simulink model "43_BusNetworkElectricityTransmissionModel"  (R2023b)
settings: Solver=VariableStepAuto  StartTime=0.0  StopTime=0.8  RelTol=1e-3
model workspace (MAT data in the model file):
  BESS_Fp_KDroop = 0.025
  BESS_KSI = 817
  BESS_PWM_fs = 560
  BESS_P_Ki = 0.5
  BESS_P_Kp = 0.0636
  BESS_Pnom = 3000000
  BESS_Q_Ki = 1
  BESS_Q_Kp = 0.0257
  BESS_Vd_Ki = 850
  BESS_Vd_Kp = 0.216
  BESS_Vnom = 1000
  BESS_Vq_KDroop = 0.025
  BESS_Vq_Ki = 850
  BESS_Vq_Kp = 0.216
  Compensation_Ki = 30
  Compensation_Kp = 3
  DC_Ki = 400
  DC_Kp = 8
  F = 0.01
  Flux_min = 0.5
  Grid_Freq_PWM = 2700
  Grid_Ireg_Ki = 5
  Grid_Ireg_Kp = 0.83
  Grid_Ireg_lim = 1.1
  Grid_Modindex_Upper = 1.1
  Grid_conv_Imax = 0.8
  H = 0.685
  Idref_max = 0.9
  Iqref_Tc = 0.3
  Ki_Var = 0.05
  Ki_Vreg = 20
  Ksh = 1.1
  L_pu = 0.3
  Llr = 0.16
  Lls = 0.18
  Lm = 2.9
  LowLoad_P = 130
  Nb_wt = 6
  P_mech = 1080000
  PeakShav_P = 200
  Pitch_Ki = 0
  Pitch_Kp = 150
  Pitch_Max = 27
  Pitch_Tc = 0.01
  Pitch_rate = 10
  Q_Filt = 50
  R_pu = 0.003
  Rotor_Freq_PWM = 1620
  Rotor_Ireg_Ki = 8
  Rotor_Ireg_Kp = 0.6
  Rotor_Ireg_lim = 0.1
  Rotor_Modindex_Upper = 2
  Rr = 0.016
  Rs = 0.023
  SOCBESS : Simulink.Parameter (value not decoded)
  T_set = 0.0001
  Tp = 5e-05
  Ts = 5e-06
  Var_C_Filt = 720000
  Var_reg_max = 1.1
  Var_reg_min = 0.9
  WT_Coeff = [0.645 116 0.4 5 21 0.00912 0.08 0.035]
  WT_H = 4.32
  WT_IGBTRon = 5.931
  WT_Param = [91.204 10143]
  Wind_Freq_Filt = 10000
  Wind_Freq_nom = 60
  Wind_P_nom = 1200000
  Wind_Rotor_V_nom = 1950
  Wind_V_nom = 500
  Zeta_Filt = 0.707106781187
  init = [-0.2 0 0 0 0 0 0 0]
  p = 3
  torque0 = 0.83
  v_Ki = 0.1
  v_Kp = 3.6
  v_Max = 1.2
  v_Min = 0.7
  v_T = 5
  vreg_max = 1
  wind_VDC_nom = 1150
  wt0 = 1.2
undefined symbols (not defined in the file): D1, D11, Delta, DiscIntNeverNeededParam, Iabc, Ion, Lithium, P, Q, Vabc
libraries: powerlib_extras x156, spsSeriesRLCBranchLib x66, spsLoadFlowBusLib x43, spsThreePhaseSeriesRLCLoadLib x33, spsThreePhaseTransformerTwoWindingsLib x32, spsThreePhaseVIMeasurementLib x30, simulink_extras x30, spsDistributedParametersLineLib x22, spsGenericPowerSystemStabilizerLib x20, spsSynchronousMachinepuStandardLib x10, spsExcitationSystemLib x10, spsHydraulicTurbineandGovernorLib x10
(part 3 of 19)

== system 43_BusNetworkElectricityTransmissionModel/North Network ==
  1320 MVar : spsThreePhaseSeriesRLCLoadLib/Three-Phase Series RLC Load  LConnTagsString=A|B|C  Configuration=Y (grounded)  NominalVoltage=650e3  Vabc=[1e3 1e3 1e3]  Vabcp=[1e3 1e3 1e3]  NominalFrequency=60  UnbalancedPower=off  ActivePower=4400e3  InductivePower=1320e6  CapacitivePower=0  Pabc=[10e3 9e3 11e3]  QLabc=[100 90 110]  QCabc=[100 90 110]  Pabcp=[10e3 9e3 11e3]  QLabcp=[100 90 110]  QCabcp=[100 90 110]  Measurements=None  LoadType=constant Z
  135 MW : spsThreePhaseSeriesRLCLoadLib/Three-Phase Series RLC Load  LConnTagsString=A|B|C  Configuration=Y (grounded)  NominalVoltage=17e3  Vabc=[1e3 1e3 1e3]  Vabcp=[1e3 1e3 1e3]  NominalFrequency=60  UnbalancedPower=off  ActivePower=135e6  InductivePower=0  CapacitivePower=0  Pabc=[10e3 9e3 11e3]  QLabc=[100 90 110]  QCabc=[100 90 110]  Pabcp=[10e3 9e3 11e3]  QLabcp=[100 90 110]  QCabcp=[100 90 110]  Measurements=None  LoadType=constant Z
  155 MW : spsThreePhaseSeriesRLCLoadLib/Three-Phase Series RLC Load  LConnTagsString=A|B|C  Configuration=Y (grounded)  NominalVoltage=17e3  Vabc=[1e3 1e3 1e3]  Vabcp=[1e3 1e3 1e3]  NominalFrequency=60  UnbalancedPower=off  ActivePower=155e6  InductivePower=0  CapacitivePower=0  Pabc=[10e3 9e3 11e3]  QLabc=[100 90 110]  QCabc=[100 90 110]  Pabcp=[10e3 9e3 11e3]  QLabcp=[100 90 110]  QCabcp=[100 90 110]  Measurements=None  LoadType=constant Z
  1980 MVar : spsThreePhaseSeriesRLCLoadLib/Three-Phase Series RLC Load  LConnTagsString=A|B|C  Configuration=Y (grounded)  NominalVoltage=650e3  Vabc=[1e3 1e3 1e3]  Vabcp=[1e3 1e3 1e3]  NominalFrequency=60  UnbalancedPower=off  ActivePower=6600e3  InductivePower=1980e6  CapacitivePower=0  Pabc=[10e3 9e3 11e3]  QLabc=[100 90 110]  QCabc=[100 90 110]  Pabcp=[10e3 9e3 11e3]  QLabcp=[100 90 110]  QCabcp=[100 90 110]  Measurements=None  LoadType=constant Z
  205 MW : spsThreePhaseSeriesRLCLoadLib/Three-Phase Series RLC Load  LConnTagsString=A|B|C  Configuration=Y (grounded)  NominalVoltage=17e3  Vabc=[1e3 1e3 1e3]  Vabcp=[1e3 1e3 1e3]  NominalFrequency=60  UnbalancedPower=off  ActivePower=205e6  InductivePower=0  CapacitivePower=0  Pabc=[10e3 9e3 11e3]  QLabc=[100 90 110]  QCabc=[100 90 110]  Pabcp=[10e3 9e3 11e3]  QLabcp=[100 90 110]  QCabcp=[100 90 110]  Measurements=None  LoadType=constant Z
  "2700 MVA 17KV :650KV Transformer " : spsThreePhaseTransformerTwoWindingsLib/Three-Phase Transformer (Two Windings)  Winding1Connection=Yg  Winding2Connection=Delta (D1)  CoreType=Three single-phase transformers  SetSaturation=off  Hysteresis=off  DataFile='hysteresis'  SetInitialFlux=off  Measurements=None  UNITS=pu  NominalPower=[ 2700e6 , 60 ]  Winding1=[650e3 , 0.002 , 0.08 ]  Winding2=[17e3 , 0.002 , 0.08 ]  Rm=500  Lm=500  L0=0.5  Saturation=[ 0,0 ; 0.0024,1.2 ; 1.0,1.52 ]  InitialFluxes=[ 0.8 , -0.8 , 0.7 ]  BreakLoop=off  DiscreteSolver=Trapezoidal iterative  DataType=off  TransfoNumber=1
  "3100 MVA 17KV :650KV Transformer " : spsThreePhaseTransformerTwoWindingsLib/Three-Phase Transformer (Two Windings)  Winding1Connection=Yg  Winding2Connection=Delta (D1)  CoreType=Three single-phase transformers  SetSaturation=off  Hysteresis=off  DataFile='hysteresis'  SetInitialFlux=off  Measurements=None  UNITS=pu  NominalPower=[ 3100e6 , 60 ]  Winding1=[ 650e3 , 0.002 , 0.08 ]  Winding2=[ 17e3 , 0.002 , 0.08 ]  Rm=500  Lm=500  L0=0.5  Saturation=[ 0,0 ; 0.0024,1.2 ; 1.0,1.52 ]  InitialFluxes=[ 0.8 , -0.8 , 0.7 ]  BreakLoop=off  DiscreteSolver=Trapezoidal iterative  DataType=off  TransfoNumber=1
  "4100 MVA 17KV :650KV Transformer " : spsThreePhaseTransformerTwoWindingsLib/Three-Phase Transformer (Two Windings)  Winding1Connection=Yg  Winding2Connection=Delta (D1)  CoreType=Three single-phase transformers  SetSaturation=off  Hysteresis=off  DataFile='hysteresis'  SetInitialFlux=off  Measurements=None  UNITS=pu  NominalPower=[ 4100e6 , 60 ]  Winding1=[ 650e3 , 0.002 , 0.08 ]  Winding2=[ 17e3 , 0.002 , 0.08 ]  Rm=500  Lm=500  L0=0.5  Saturation=[ 0,0 ; 0.0024,1.2 ; 1.0,1.52 ]  InitialFluxes=[ 0.8 , -0.8 , 0.7 ]  BreakLoop=off  DiscreteSolver=Trapezoidal iterative  DataType=off  TransfoNumber=1
  660 MVar : spsThreePhaseSeriesRLCLoadLib/Three-Phase Series RLC Load  LConnTagsString=A|B|C  Configuration=Y (grounded)  NominalVoltage=650e3  Vabc=[1e3 1e3 1e3]  Vabcp=[1e3 1e3 1e3]  NominalFrequency=60  UnbalancedPower=off  ActivePower=2200e3  InductivePower=660e6  CapacitivePower=0  Pabc=[10e3 9e3 11e3]  QLabc=[100 90 110]  QCabc=[100 90 110]  Pabcp=[10e3 9e3 11e3]  QLabcp=[100 90 110]  QCabcp=[100 90 110]  Measurements=None  LoadType=constant Z
  990 Mvar : spsThreePhaseParallelRLCLoadLib/Three-Phase Parallel RLC Load  LConnTagsString=A|B|C  Configuration=Y (grounded)  NominalVoltage=650e3  Vabc=[1e3 1e3 1e3]  Vabcp=[1e3 1e3 1e3]  NominalFrequency=60  UnbalancedPower=off  ActivePower=3300e3  InductivePower=990e6  CapacitivePower=0  Pabc=[10e3 9e3 11e3]  QLabc=[100 90 110]  QCabc=[100 90 110]  Pabcp=[10e3 9e3 11e3]  QLabcp=[100 90 110]  QCabcp=[100 90 110]  Measurements=None  LoadType=constant Z
  ATL-CAD 447 km : spsDistributedParametersLineLib/Distributed Parameters Line  Phases=3  Length=447  Frequency=60  Resistance=[0.01273 0.3864]/6  Inductance="[0.9337e-3  4.1264e-3]/6"  Capacitance=[12.74e-9 7.751e-9]*6  x1=[-0.00258 -1.67008857282466e-09 -194881.82529365 -120209.574728766;-0.00252 -2.05415012980081e-09 -192113.110957955 -124586.590676799;-0.00246 -2.43716074561422e-09 -189246.108004852 -128899.865822947;-0.0024 -2.81892446495662e-09 -186282.283246028 -133147.193415944;-0.00234 -3.19924597045502e-09 -183223.153028994 -137326.400444512;-0.00228 -3.57793068259966e-09 -180070.282461296 -141435.348749113;-0.00222 -3.95478485929453e-09 -176825.284609774 -145471.936115869;-0.00216 -4.32961569497935e-09 -173489.819675291 -149434.097352096;-0.0021 -4.70223141927253e-09 -170065.594143338 -153319.805342892;-0.00204 -5.07244139508436e-09 -166554.359910971 -157127.072088251;-0.00198 -5.44005621615053e-09 -162957.913390503 -160853.949720156;-0.00192 -5.80488780393583e-09 -159278.094590428 -164498.531499144;-0.00186 -6.16674950385864e-09 -155516.78617404 -168058.952789834;-0.0018 -6.52545618078685e-09 -151675.912496225 -171533.392014904;-0.00174 -6.88082431375641e-09 -147757.438618928 -174920.071587046;-0.00168 -7.23267208986403e-09 -143763.369305791 -178217.258818414;-0.00162 -7.58081949728606e-09 -139695.747996475 -181423.266807093;-0.00156 -7.92508841737585e-09 -135556.655761204 -184536.455300158;-0.0015 -8.2653027157925e-09 -131348.210236046 -187555.231532849;-0.00144 -8.60128833261452e-09 -127072.564539495 -190478.051043466;-0.00138 -8.93287337139205e-09 -122731.906170895 -193303.41846354;-0.00132 -9.25988818709224e-09 -118328.455891273 -196029.88828289;-0.00126 -9.58216547289286e-09 -113864.466587159 -198656.06558918;-0.0012 -9.89954034577949e-09 -109342.222117965 -201180.606781572;-0.00114 -1.02118504309027e-08 -104764.036147524 -203602.220258145;-0.00108 -1.05189359446522e-08 -100132.250960373 -205919.667076697;-0.00102 -1.08206397764049e-08 -95449.2362633992 -208131.761588614;-0.00096 -1.11168075689055e-08 -90717.387973454 -210237.37204547;-0.0009 -1.14072877972388e-08 -85939.126991557 -212235.421178048;-0.00084 -1.16919318463526e-08 -81116.8979643186 -214124.886747491;-0.00078 -1.19705940870918e-08 -76253.1680332137 -215904.802068301;-0.00072 -1.22431319507049e-08 -71350.4255723465 -217574.256502911;-0.00066 -1.25094060017849e-08 -66411.1789153522 -219132.395927584;-0.0006 -1.27692800096072e-08 -61437.9550720873 -220578.423169399;-0.00054 -1.30226210178274e-08 -56433.2984357647 -221911.598414101;-0.00048 -1.32692994125045e-08 -51399.7694811948 -223131.239584599;-0.00042 -1.35091889884137e-08 -46339.9434547999 -224236.722689934;-0.00036 -1.37421670136153e-08 -41256.4090570697 -225227.482144522;-0.0003 -1.39681142922467e-08 -36151.7671181352 -226103.01105752;-0.00024 -1.41869152255051e-08 -31028.6292671352 -226862.861492158;-0.00018 -1.43984578707901e-08 -25889.616596059 -227506.644694913;-0.00012 -1.46026339989755e-08 -20737.3583187471 -228034.031294402;-6e-05 -1.47993391497814e-08 -15574.490425737 -228444.751469897]  x2=[-0.00258 5.15041171457139e-09 -301593.332748427 -116993.562625722;-0.00252 4.92493877262698e-09 -298870.048576722 -123784.957337496;-0.00246 4.69694614100409e-09 -295993.856965682 -130513.021377814;-0.0024 4.46655046494587e-09 -292966.22942808 -137174.312544791;-0.00234 4.23386961913743e-09 -289788.714954109 -143765.422798781;-0.00228 3.99902264739891e-09 -286462.939218889 -150282.980005987;-0.00222 3.76212970178055e-09 -282990.603750737 -156723.649663712;-0.00216 3.52331198109059e-09 -279373.485060641 -163084.136606349;-0.0021 3.28269166888779e-09 -275613.43373336 -169361.186691249;-0.00204 3.04039187097001e-09 -271712.37348063 -175551.588463604;-0.00198 2.79653655239106e-09 -267672.30015696 -181652.17479948;-0.00192 2.55125047403786e-09 -263495.280738514 -187659.824526183;-0.00186 2.30465912880045e-09 -259183.45226561 -193571.464019103;-0.0018 2.05688867736754e-09 -254739.020749366 -199384.068774241;-0.00174 1.80806588368036e-09 -250164.260043072 -205094.664955601;-0.00168 1.55831805007787e-09 -245461.510678835 -210700.330916655;-0.00162 1.30777295216655e-09 -240633.178670128 -216198.198695118;-0.00156 1.05655877344804e-09 -235681.734280824 -221585.455480246;-0.0015 8.04804039738072e-10 -230609.710761363 -226859.345051921;-0.00144 5.52637553410304e-10 -225419.7030527 -232017.169190789;-0.00138 3.00188327498644e-10 -220114.366458677 -237056.289058714;-0.00132 4.75855196917949e-11 -214696.415287529 -241974.126548861;-0.00126 -2.05041633746211e-10 -209168.621463186 -246768.165604697;-0.0012 -4.57563884095657e-10 -203533.81310711 -251435.953507259;-0.00114 -7.0985203630719e-10 -197794.873091376 -255975.102130004;-0.00108 -9.61777015100393e-10 -191954.73756374 -260383.289160623;-0.00102 -1.21320993100107e-09 -186016.394445451 -264658.259289177;-0.00096 -1.46402214628351e-09 -179982.881902575 -268797.825361957;-0.0009 -1.71408534078389e-09 -173857.286791617 -272799.869500469;-0.00084 -1.96327157755127e-09 -167642.743080223 -276662.344184983;-0.00078 -2.21145336830249e-09 -161342.430243787 -280383.273302079;-0.00072 -2.45850373864752e-09 -154959.571638773 -283960.753155667;-0.00066 -2.70429629305194e-09 -148497.432853586 -287392.953440949;-0.0006 -2.94870527950318e-09 -141959.320037833 -290678.118180839;-0.00054 -3.19160565384762e-09 -135348.578210842 -293814.566624354;-0.00048 -3.43287314376546e-09 -128668.589550285 -296800.694106514;-0.00042 -3.67238431235074e-09 -121922.771661791 -299634.972869324;-0.00036 -3.91001662126397e-09 -115114.575830441 -302315.952843396;-0.0003 -4.14564849342495e-09 -108247.485255024 -304842.262389837;-0.00024 -4.37915937521393e-09 -101325.013265967 -307212.609002002;-0.00018 -4.61042979814898e-09 -94350.7015278514 -309425.779966765;-0.00012 -4.83934144000835e-09 -87328.118227434 -311480.642984966;-6e-05 -5.06577718536627e-09 -80260.8562480934 -313376.146750715]  x3=[-0.00258 5.51282931221187e-12 -5052.77243318941 2918.73418538423;-0.00252 4.31538249983226e-12 -5117.49377650402 2803.70636456851;-0.00246 3.11572785802664e-12 -5179.59691544217 2687.24411577014;-0.0024 1.91447915227681e-12 -5239.05007689043 2569.40702322757;-0.00234 7.12250963617166e-13 -5295.82284351283 2450.25537457474;-0.00228 -4.90341625796339e-13 -5349.88616931294 2329.85012999677;-0.00222 -1.69268334737362e-12 -5401.2123944943 2208.2528910416;-0.00216 -2.89415906087319e-12 -5449.77525961171 2085.52586910356;-0.0021 -4.09415406911931e-12 -5495.54991900603 1961.7318535948;-0.00204 -5.29205443249241e-12 -5538.5129535157 1836.9341798211;-0.00198 -6.48724728303191e-12 -5578.6423824584 1711.19669657837;-0.00192 -7.67912113799086e-12 -5615.91767487677 1584.58373348638;-0.00186 -8.86706621268178e-12 -5650.31976004245 1457.1600680766;-0.0018 -1.00504747324537e-11 -5681.83103721298 1328.99089265078;-0.00174 -1.12287412436412e-11 -5710.43538463672 1200.14178092734;-0.00168 -1.2401262923325e-11 -5736.11816780095 1070.67865449271;-0.00162 -1.35674398877484e-11 -5758.86624691927 940.66774907458;-0.00156 -1.47266754992277e-11 -5778.66798365404 810.175580654477;-0.0015 -1.58783766714039e-11 -5795.51324707088 679.268911436989;-0.00144 -1.70219541726763e-11 -5809.39341882173 548.014715692963;-0.00138 -1.81568229276645e-11 -5820.30139755427 416.480145494241;-0.00132 -1.92824023165433e-11 -5828.23160254502 284.732496357416;-0.00126 -2.03981164720992e-11 -5833.17997655457 152.839172814202;-0.0012 -2.15033945743541e-11 -5835.14398790334 20.8676539260338;-0.00114 -2.25976711426077e-11 -5834.12263176683 -111.114541239473;-0.00108 -2.36803863247478e-11 -5830.11643068972 -243.039888152521;-0.00102 -2.4750986183681e-11 -5823.12743431851 -374.840891367929;-0.00096 -2.58089229807369e-11 -5813.15921835287 -506.450119057049;-0.0009 -2.68536554559018e-11 -5800.2168827163 -637.800237507139;-0.00084 -2.7884649104737e-11 -5784.30704894683 -768.824045570526;-0.00078 -2.89013764518411e-11 -5765.43785680943 -899.454509045965;-0.00072 -2.99033173207164e-11 -5743.61896013143 -1029.62479497457;-0.00066 -3.08899590999007e-11 -5718.86152186356 -1159.26830583278;-0.0006 -3.18607970052286e-11 -5691.17820836869 -1288.31871360492;-0.00054 -3.28153343380888e-11 -5660.58318294154 -1416.70999371778;-0.00048 -3.3753082739544e-11 -5627.09209856244 -1544.37645882006;-0.00042 -3.46735624401844e-11 -5590.72208988901 -1671.25279238922;-0.00036 -3.55763025055866e-11 -5551.49176448973 -1797.27408214859;-0.0003 -3.64608410772525e-11 -5509.42119332396 -1922.37585327772;-0.00024 -3.73267256089044e-11 -5464.53190047329 -2046.4941013989;-0.00018 -3.81735130980161e-11 -5416.8468521294 -2169.56532532294;-0.00012 -3.90007703124615e-11 -5366.39044484413 -2291.52655953759;-6e-05 -3.98080740121637e-11 -5313.18849304779 -2412.31540642183]  x4=[-0.00258 1.21970167270157e-10 -7329.45055634832 -4834.93116395816;-0.00252 1.19241005783673e-10 -7218.22081108888 -4999.4692217727;-0.00246 1.1645083839531e-10 -7103.29809068509 -5161.44945875382;-0.0024 1.1360109260626e-10 -6984.74119172425 -5320.78900281922;-0.00234 1.10693226399125e-10 -6862.61077010654 -5477.40633291389;-0.00228 1.0772872749199e-10 -6736.96931001239 -5631.22132071782;-0.00222 1.04709112577271e-10 -6607.88109193435 -5782.15527164106;-0.00216 1.01635926545756e-10 -6475.41215979007 -5930.13096508538;-0.0021 9.85107416962035e-11 -6339.63028713298 -6075.07269395175;-0.00204 9.53351569309305e-11 -6200.6049424781 -6216.90630337345;-0.00198 9.21107969377804e-11 -6058.40725376064 -6355.55922865513;-0.00192 8.88393113589052e-11 -5913.10997194567 -6490.96053239819;-0.00186 8.5522373946777e-11 -5764.78743380733 -6623.04094079372;-0.0018 8.21616817078658e-11 -5613.51552389683 -6751.73287906421;-0.00174 7.87589540344196e-11 -5459.37163571847 -6876.9705060361;-0.00168 7.53159318247913e-11 -5302.43463213369 -6998.68974782529;-0.00162 7.18343765927629e-11 -5142.78480501338 -7116.82833061858;-0.00156 6.8316069566323e-11 -4980.50383415909 -7231.32581253405;-0.0015 6.47628107763572e-11 -4815.67474551411 -7342.1236145443;-0.00144 6.11764181357191e-11 -4648.38186868589 -7449.16505044649;-0.00138 5.75587265091524e-11 -4478.71079380142 -7552.39535586414;-0.00132 5.39115867745408e-11 -4306.74832771779 -7651.76171626551;-0.00126 5.02368648759636e-11 -4132.58244961014 -7747.21329398453;-0.0012 4.65364408690454e-11 -3956.30226595993 -7838.70125423031;-0.00114 4.2812207959084e-11 -3777.99796496638 -7926.17879007188;-0.00108 3.90660715324522e-11 -3597.76077040459 -8009.6011463855;-0.00102 3.52999481817663e-11 -3415.68289495368 -8088.92564275222;-0.00096 3.15157647253225e-11 -3231.85749301915 -8164.11169529394;-0.0009 2.7715457221301e-11 -3046.37861307333 -8235.12083743692;-0.00084 2.39009699772422e-11 -2859.34114953846 -8301.91673959193;-0.00078 2.00742545553039e-11 -2670.84079423694 -8364.46522774117;-0.00072 1.62372687738056e-11 -2480.97398743362 -8422.73430092236;-0.00066 1.23919757055724e-11 -2289.8378684952 -8476.69414760096;-0.0006 8.54034267359075e-12 -2097.53022619192 -8526.31716092235;-0.00054 4.68434024448995e-12 -1904.14944866701 -8571.57795283598;-0.00048 8.25941220363423e-13 -1709.79447309954 -8612.4533670844;-0.00042 -3.03288037055309e-12 -1514.56473508625 -8648.92249105037;-0.00036 -6.89015028383084e-12 -1318.56011776856 -8680.9666664562;-0.0003 -1.0743895068908e-11 -1121.88090073043 -8708.56949890966;-0.00024 -1.45921430787436e-11 -924.627708693503 -8731.71686629162;-0.00018 -1.84329254785483e-11 -726.901460035657 -8750.3969259812;-0.00012 -2.22642772530769e-11 -528.803315159263 -8764.6001209147;-6e-05 -2.60842382119663e-11 -330.434624735671 -8774.31918447516]  x5=0.00252797080447097  V1=[6.404e-19 2.341e-08 2.341e-08;377 377 377;-1.588 0.8733 -0.6975]  V2=[3.447e-16 8.016e-05 8.016e-05;377 377 377;2.581 0.8892 -0.6816]  I1=[4.995e-19 5.332e-07 5.332e-07;377 377 377;1.203 -0.6479 -2.219]  I2=[4.022e-19 5.225e-07 5.225e-07;377 377 377;-2.95 1.909 0.3385]  nHarmo=1  Measurements=None  Decoupling=off  VsMag0=0  VrMag0=0  VsAngle0=0  VrAngle0=0  IsMag0=0  IrMag0=0  IsAngle0=0  IrAngle0=0
      settings: LibrarySourceBlock=sps_lib/Power Grid Elements/Distributed Parameters Line
  BMW 1 : spsThreePhaseVIMeasurementLib/Three-Phase V-I Measurement  VoltageMeasurement=no  SetLabelV=off  LabelV=Vabc  Vpu=off  VpuLL=off  CurrentMeasurement=no  SetLabelI=off  LabelI=Iabc  Ipu=off  Pbase=100e6  Vbase=500e3  OutputType=Complex  PhasorSimulation=off  PSBequivalent=0
  BMW- FER 131 km : spsDistributedParametersLineLib/Distributed Parameters Line  Phases=3  Length=131  Frequency=60  Resistance=[0.01273 0.3864]/6  Inductance="[0.9337e-3  4.1264e-3]/6"  Capacitance=[12.74e-9 7.751e-9]*6  x1=[-0.00078 -1.19705940870918e-08 -76253.1680332137 -215904.802068301;-0.00072 -1.22431319507049e-08 -71350.4255723465 -217574.256502911;-0.00066 -1.25094060017849e-08 -66411.1789153522 -219132.395927584;-0.0006 -1.27692800096072e-08 -61437.9550720873 -220578.423169399;-0.00054 -1.30226210178274e-08 -56433.2984357647 -221911.598414101;-0.00048 -1.32692994125045e-08 -51399.7694811948 -223131.239584599;-0.00042 -1.35091889884137e-08 -46339.9434547999 -224236.722689934;-0.00036 -1.37421670136153e-08 -41256.4090570697 -225227.482144522;-0.0003 -1.39681142922467e-08 -36151.7671181352 -226103.01105752;-0.00024 -1.41869152255051e-08 -31028.6292671352 -226862.861492158;-0.00018 -1.43984578707901e-08 -25889.616596059 -227506.644694913;-0.00012 -1.46026339989755e-08 -20737.3583187471 -228034.031294402;-6e-05 -1.47993391497814e-08 -15574.490425737 -228444.751469897]  x2=[-0.00078 -1.84679215935695e-10 -40323.6266116141 -194988.996299748;-0.00072 2.82824148749058e-10 -35903.1411858874 -195851.159993976;-0.00066 7.50182815373322e-10 -31464.2870497162 -196613.122615838;-0.0006 1.21715767460746e-09 -27009.3352028971 -197274.494331177;-0.00054 1.68350981348478e-09 -22540.5648811132 -197834.936770003;-0.00048 2.14900063763383e-09 -18060.2623898343 -198294.163199608;-0.00042 2.6133919933477e-09 -13570.7199346015 -198651.938671265;-0.00036 3.07644628942785e-09 -9074.23444829206 -198908.080140432;-0.0003 3.53792661874013e-09 -4573.10641596632 -199062.456560401;-0.00024 3.9975968794209e-09 -69.6386978968809 -199114.988949342;-0.00018 4.45522189567106e-09 4433.86464861718 -199065.650430714;-0.00012 4.91056753807636e-09 8935.09954804861 -198914.466247016;-6e-05 5.36340084339233e-09 13431.7630854496 -198661.513746869]  x3=[-0.00078 -8.93963344042616e-10 801.480589851872 -9198.62669723828;-0.00072 -8.84038389071924e-10 1009.32547419504 -9178.14688538209;-0.00066 -8.73661143726232e-10 1216.65396897542 -9152.97136398669;-0.0006 -8.62836917196007e-10 1423.36000110408 -9123.11301331401;-0.00054 -8.51571247355552e-10 1629.33781595552 -9088.58710944798;-0.00048 -8.39869897929723e-10 1834.48203147361 -9049.41131647897;-0.00042 -8.27738855545101e-10 2038.68769208707 -9005.60567746655;-0.00036 -8.15184326667126e-10 2241.85032240664 -8957.19260418508;-0.0003 -8.02212734424755e-10 2443.86598067664 -8904.19686565742;-0.00024 -7.88830715324265e-10 2644.63131195347 -8846.64557548264;-0.00018 -7.75045115853899e-10 2844.04360098393 -8784.56817796424;-0.00012 -7.60862988981075e-10 3042.00082475626 -8717.99643304583;-6e-05 -7.46291590543957e-10 3238.40170469692 -8646.96440006223]  x4=[-0.00078 7.88145612187523e-10 -4148.32191911194 353.877291066962;-0.00072 7.79406939715943e-10 -4155.2640953326 259.961667664255;-0.00066 7.7026950825222e-10 -4160.08036166163 165.913043068831;-0.0006 7.60737992675131e-10 -4162.76825400819 71.7795342948529;-0.00054 7.50817269484168e-10 -4163.32639719688 -22.3906982152036;-0.00048 7.40512414304629e-10 -4161.75450567134 -116.549475230321;-0.00042 7.29828699290835e-10 -4158.05338364032 -210.648623380323;-0.00036 7.187715904288e-10 -4152.22492466623 -304.639999802266;-0.0003 7.0734674473973e-10 -4144.27211069639 -398.475516771209;-0.00024 6.95560007385786e-10 -4134.19901053738 -492.107166302792;-0.00018 6.83417408679592e-10 -4122.01077777336 -585.487044714998;-0.00012 6.70925160999016e-10 -4107.71364812942 -678.567377136572;-6e-05 6.58089655608801e-10 -4091.31493628129 -771.30054194952]  x5=0.000740859452764423  V1=[1.271e-18 2.341e-08 2.341e-08;377 377 377;2.226 1.284 -0.2866]  V2=[3.351e-20 3.07e-09 3.07e-09;377 377 377;-0.6702 -1.817 2.896]  I1=[5.66e-21 5.705e-10 5.705e-10;377 377 377;-2.518 2.745 1.174]  I2=[6.071e-21 5.74e-10 5.74e-10;377 377 377;0.8934 -0.2657 -1.836]  nHarmo=1  Measurements=None  Decoupling=off  VsMag0=0  VrMag0=0  VsAngle0=0  VrAngle0=0  IsMag0=0  IrMag0=0  IsAngle0=0  IrAngle0=0
      settings: LibrarySourceBlock=sps_lib/Power Grid Elements/Distributed Parameters Line
  BMW- ORE 215 km : spsDistributedParametersLineLib/Distributed Parameters Line  Phases=3  Length=215  Frequency=60  Resistance=[0.01273 0.3864]/6  Inductance="[0.9337e-3  4.1264e-3]/6"  Capacitance=[12.74e-9 7.751e-9]*6  x1=[-0.00126 -9.58216547289286e-09 -113864.466587159 -198656.06558918;-0.0012 -9.89954034577949e-09 -109342.222117965 -201180.606781572;-0.00114 -1.02118504309027e-08 -104764.036147524 -203602.220258145;-0.00108 -1.05189359446522e-08 -100132.250960373 -205919.667076697;-0.00102 -1.08206397764049e-08 -95449.2362633992 -208131.761588614;-0.00096 -1.11168075689055e-08 -90717.387973454 -210237.37204547;-0.0009 -1.14072877972388e-08 -85939.126991557 -212235.421178048;-0.00084 -1.16919318463526e-08 -81116.8979643186 -214124.886747491;-0.00078 -1.19705940870918e-08 -76253.1680332137 -215904.802068301;-0.00072 -1.22431319507049e-08 -71350.4255723465 -217574.256502911;-0.00066 -1.25094060017849e-08 -66411.1789153522 -219132.395927584;-0.0006 -1.27692800096072e-08 -61437.9550720873 -220578.423169399;-0.00054 -1.30226210178274e-08 -56433.2984357647 -221911.598414101;-0.00048 -1.32692994125045e-08 -51399.7694811948 -223131.239584599;-0.00042 -1.35091889884137e-08 -46339.9434547999 -224236.722689934;-0.00036 -1.37421670136153e-08 -41256.4090570697 -225227.482144522;-0.0003 -1.39681142922467e-08 -36151.7671181352 -226103.01105752;-0.00024 -1.41869152255051e-08 -31028.6292671352 -226862.861492158;-0.00018 -1.43984578707901e-08 -25889.616596059 -227506.644694913;-0.00012 -1.46026339989755e-08 -20737.3583187471 -228034.031294402;-6e-05 -1.47993391497814e-08 -15574.490425737 -228444.751469897]  x2=[-0.00126 6.50309734918414e-09 -202799.306931214 -207001.083285656;-0.0012 5.98047046812839e-09 -198065.563080492 -211534.981265528;-0.00114 5.45478386787474e-09 -193230.485227868 -215960.654040268;-0.00108 4.92630649940148e-09 -188296.547088512 -220275.837353906;-0.00102 4.39530874149545e-09 -183266.272956345 -224478.323478925;-0.00096 3.8620622624213e-09 -178142.236412563 -228565.962345769;-0.0009 3.32683988093099e-09 -172927.059008942 -232536.662642864;-0.00084 2.78991542668466e-09 -167623.408926607 -236388.392886568;-0.00078 2.25156360015433e-09 -162233.999610941 -240119.182460515;-0.00072 1.71205983208205e-09 -156761.588383335 -243727.122623823;-0.00066 1.17168014256445e-09 -151208.97503049 -247210.367487638;-0.0006 6.30700999835754e-10 -145579.000371999 -250567.134959523;-0.00054 8.93991788215252e-11 -139874.544806927 -253795.707655215;-0.00048 -4.51948380464494e-10 -134098.526840148 -256894.433777264;-0.00042 -9.93064714608022e-10 -128253.901589181 -259861.72796013;-0.00036 -1.53367297849383e-09 -122343.659272302 -262696.072081279;-0.0003 -2.07349658694482e-09 -116370.823678688 -265396.016037886;-0.00024 -2.61225935622812e-09 -110338.450621394 -267960.178488734;-0.00018 -3.14968564535578e-09 -104249.626373943 -270387.247560931;-0.00012 -3.68550049710776e-09 -98107.4660913263 -272675.981521095;-6e-05 -4.21942977870521e-09 -91915.1122162403 -274825.20941064]  x3=[-0.00126 1.65771973171058e-10 -4039.34540789377 3058.66441287293;-0.0012 1.6818222170819e-10 -4107.490998384 2966.52179794441;-0.00114 1.70506425113046e-10 -4173.53512058175 2872.86145564905;-0.00108 1.72743394280217e-10 -4237.44398509375 2777.7313043486;-0.00102 1.74891984734944e-10 -4299.18489496401 2681.18001438628;-0.00096 1.76951097218648e-10 -4358.72626240221 2583.25698318608;-0.0009 1.78919678251335e-10 -4416.03762494456 2484.01230998018;-0.00084 1.80796720670572e-10 -4471.08966103899 2383.49677017723;-0.00078 1.82581264146776e-10 -4523.8542050466 2281.7617893847;-0.00072 1.84272395674528e-10 -4574.3042616517 2178.85941709861;-0.00066 1.8586925003969e-10 -4622.41401967311 2074.84230007404;-0.0006 1.87371010262064e-10 -4668.15886526966 1969.76365539007;-0.00054 1.88776908013369e-10 -4711.51539453308 1863.67724322296;-0.00048 1.90086224010338e-10 -4752.46142546187 1756.63733934142;-0.00042 1.91298288382714e-10 -4790.97600931 1648.69870733815;-0.00036 1.92412481015967e-10 -4827.0394413047 1539.91657061175;-0.0003 1.93428231868559e-10 -4860.6332707278 1430.34658411344;-0.00024 1.94345021263584e-10 -4891.74031035543 1320.04480587294;-0.00018 1.95162380154648e-10 -4920.3446452513 1209.06766831812;-0.00012 1.95879890365838e-10 -4946.43164090915 1097.47194940319;-6e-05 1.96497184805673e-10 -4969.98795073996 985.31474356]  x4=[-0.00126 -1.20908843861436e-10 -4184.12959328111 -10998.5446924139;-0.0012 -1.29836564733162e-10 -3934.2992777039 -11090.3669013412;-0.00114 -1.38697858819266e-10 -3682.45610191872 -11176.5150736354;-0.00108 -1.47488192517956e-10 -3428.72891354783 -11256.9451342996;-0.00102 -1.56203068532086e-10 -3173.24752410915 -11331.6159338286;-0.00096 -1.64838028170054e-10 -2916.14264260226 -11400.4892692618;-0.0009 -1.73388653626954e-10 -2657.54580863529 -11463.529903728;-0.00084 -1.81850570244804e-10 -2397.58932512683 -11520.7055844737;-0.00078 -1.90219448750705e-10 -2136.40619061727 -11571.9870593643;-0.00072 -1.98491007471773e-10 -1874.13003122435 -11617.3480918495;-0.00066 -2.06661014525727e-10 -1610.89503227751 -11656.7654743871;-0.0006 -2.14725289985993e-10 -1346.83586966624 -11690.2190403157;-0.00054 -2.22679708020235e-10 -1082.08764093738 -11717.6916741728;-0.00048 -2.30520199001206e-10 -816.785796176738 -11739.1693204514;-0.00042 -2.38242751588845e-10 -551.066068710306 -11754.6409907908;-0.00036 -2.4584341478255e-10 -285.064405660592 -11764.0987695985;-0.0003 -2.53318299942589e-10 -18.9168983935577 -11767.5378181001;-0.00024 -2.60663582779593e-10 247.240287108239 -11764.9563768148;-0.00018 -2.67875505311138e-10 513.270979910676 -11756.3557664558;-0.00012 -2.74950377784396e-10 779.039073795634 -11741.7403872542;-6e-05 -2.8188458056388e-10 1044.40859689545 -11721.117716708]  x5=0.00121591436904085  V1=[1.271e-18 2.341e-08 2.341e-08;377 377 377;2.047 1.175 -0.3959]  V2=[2.813e-15 0.004697 0.004697;377 377 377;-0.9882 1.143 -0.4279]  I1=[7.991e-18 6.252e-05 6.252e-05;377 377 377;-2.327 -0.3924 -1.963]  I2=[7.132e-18 6.19e-05 6.19e-05;377 377 377;0.3426 2.469 0.8982]  nHarmo=1  Measurements=None  Decoupling=off  VsMag0=0  VrMag0=0  VsAngle0=0  VrAngle0=0  IsMag0=0  IrMag0=0  IsAngle0=0  IrAngle0=0
      settings: LibrarySourceBlock=sps_lib/Power Grid Elements/Distributed Parameters Line
  CAD 3 : spsThreePhaseVIMeasurementLib/Three-Phase V-I Measurement  VoltageMeasurement=no  SetLabelV=off  LabelV=Vabc  Vpu=off  VpuLL=off  CurrentMeasurement=no  SetLabelI=off  LabelI=Iabc  Ipu=off  Pbase=100e6  Vbase=500e3  OutputType=Complex  PhasorSimulation=off  PSBequivalent=0
  Cs BMW- MPP8 : Subsystem
  Cs BMWN : Subsystem
  Cs FER : Subsystem
  Cs LTNN : Subsystem
  Cs ORED : Subsystem
  FER-LTN 78 km : spsDistributedParametersLineLib/Distributed Parameters Line  Phases=3  Length=78  Frequency=60  Resistance=[0.01273 0.3864]/6  Inductance="[0.9337e-3  4.1264e-3]/6"  Capacitance=[12.74e-9 7.751e-9]*6  x1=[-0.00048 -1.16937399343794e-09 0 0;-0.00042 -7.96828963434923e-10 0 0;-0.00036 -4.23876261010511e-10 0 0;-0.0003 -5.07066956586323e-11 -25934.923705434 -220693.628977832;-0.00024 3.22488812175697e-10 -20936.7468426592 -221223.782464588;-0.00018 6.95519328774809e-10 -15927.8583533331 -221640.753776489;-0.00012 1.0681940048336e-09 -10910.8208773604 -221944.329583308;-6e-05 1.44032217310156e-09 -5888.20122381812 -222134.354570052]  x2=[-0.00048 7.78041349050393e-09 0 0;-0.00042 8.5731532508491e-09 0 0;-0.00036 9.36150682757748e-09 0 0;-0.0003 1.01450708844321e-08 -7150.14822079248 -204050.585017666;-0.00024 1.09234445355629e-08 -2533.20208774904 -204160.128306381;-0.00018 1.16962295506273e-08 2085.04007829069 -204165.219501008;-0.00012 1.24630305585321e-08 6702.21549929925 -204065.855996799;-6e-05 1.32234552497128e-08 11315.9619430157 -203862.088629959]  x3=[-0.00048 -7.75649349725857e-10 0 0;-0.00042 -7.58329745316695e-10 0 0;-0.00036 -7.40622165397507e-10 0 0;-0.0003 -7.22535669493377e-10 2958.82173994833 -8816.93119537568;-0.00024 -7.0407951098981e-10 3157.48156193806 -8747.75517282301;-0.00018 -6.85263132398528e-10 3354.52595801715 -8674.10363708399;-0.00012 -6.66096160526503e-10 3549.8541166316 -8596.01426964524;-6e-05 -6.46588401550711e-10 3743.36610428622 -8513.52702247006]  x4=[-0.00048 8.01840901977148e-10 0 0;-0.00042 7.94117538895057e-10 0 0;-0.00036 7.85987890606462e-10 0 0;-0.0003 7.77456116389647e-10 -4166.96813804089 -533.728222533507;-0.00024 7.68526581257949e-10 -4153.83015319847 -627.838614952894;-0.00018 7.59203853726542e-10 -4138.56699209571 -721.627793535747;-0.00012 7.49492703475093e-10 -4121.18646364787 -815.047774005279;-6e-05 7.39398098907514e-10 -4101.69746005446 -908.050760973279]  x5=0.000441122422256679  V1=[6.391e-24 5.815e-13 5.815e-13;377 377 377;2.579 1.39 -0.1804]  V2=[2.845e-25 1.398e-13 1.398e-13;377 377 377;-0.3188 -1.706 3.006]  I1=[5.031e-26 2.613e-14 2.613e-14;377 377 377;-2.041 2.924 1.353]  I2=[5.244e-26 2.622e-14 2.622e-14;377 377 377;1.254 -0.1553 -1.726]  nHarmo=1  Measurements=None  Decoupling=off  VsMag0=0  VrMag0=0  VsAngle0=0  VrAngle0=0  IsMag0=0  IrMag0=0  IsAngle0=0  IrAngle0=0
      settings: LibrarySourceBlock=sps_lib/Power Grid Elements/Distributed Parameters Line
  LTN 3 : spsThreePhaseVIMeasurementLib/Three-Phase V-I Measurement  VoltageMeasurement=no  SetLabelV=off  LabelV=Vabc  Vpu=off  VpuLL=off  CurrentMeasurement=no  SetLabelI=off  LabelI=Iabc  Ipu=off  Pbase=100e6  Vbase=500e3  OutputType=Complex  PhasorSimulation=off  PSBequivalent=0
  Load Flow Bus : spsLoadFlowBusLib/Load Flow Bus  LConnTagsString=a  Phases=single  Connectors=on one side  ID=BUS_13  Vbase=17e3  Vref=1  Vangle=0  VLF=1  VLFb=1  VLFc=1  angleLF=0  angleLFb=0  angleLFc=0
  Load Flow Bus1 : spsLoadFlowBusLib/Load Flow Bus  LConnTagsString=a  Phases=single  Connectors=on one side  ID=BUS_14  Vbase=650e3  Vref=1  Vangle=0  VLF=1  VLFb=1  VLFc=1  angleLF=0  angleLFb=0  angleLFc=0
  Load Flow Bus2 : spsLoadFlowBusLib/Load Flow Bus  LConnTagsString=a  Phases=single  Connectors=on one side  ID=BUS_15  Vbase=17e3  Vref=1  Vangle=0  VLF=1  VLFb=1  VLFc=1  angleLF=0  angleLFb=0  angleLFc=0
  Load Flow Bus3 : spsLoadFlowBusLib/Load Flow Bus  LConnTagsString=a  Phases=single  Connectors=on one side  ID=BUS_16  Vbase=650e3  Vref=1  Vangle=0  VLF=1  VLFb=1  VLFc=1  angleLF=0  angleLFb=0  angleLFc=0
  Load Flow Bus4 : spsLoadFlowBusLib/Load Flow Bus  LConnTagsString=a  Phases=single  Connectors=on one side  ID=BUS_17  Vbase=17e3  Vref=1  Vangle=0  VLF=1  VLFb=1  VLFc=1  angleLF=0  angleLFb=0  angleLFc=0
  Load Flow Bus6 : spsLoadFlowBusLib/Load Flow Bus  LConnTagsString=a  Phases=single  Connectors=on one side  ID=BUS_18  Vbase=650e3  Vref=1  Vangle=0  VLF=1  VLFb=1  VLFc=1  angleLF=0  angleLFb=0  angleLFc=0
  Load Flow Bus7 : spsLoadFlowBusLib/Load Flow Bus  LConnTagsString=a  Phases=single  Connectors=on one side  ID=BUS_19  Vbase=650e3  Vref=1  Vangle=0  VLF=1  VLFb=1  VLFc=1  angleLF=0  angleLFb=0  angleLFc=0
  Load Flow Bus8 : spsLoadFlowBusLib/Load Flow Bus  LConnTagsString=a  Phases=single  Connectors=on one side  ID=BUS_20  Vbase=650e3  Vref=1  Vangle=0  VLF=1  VLFb=1  VLFc=1  angleLF=0  angleLFb=0  angleLFc=0
  MPP7 2700 MVA 17KV : spsSynchronousMachinepuStandardLib/Synchronous Machine pu Standard  PresetModel=No  MechanicalLoad=Mechanical power Pm  ShowDetailedParameters=on  RotorType=Salient-pole  Units=per unit standard parameters  MeasurementBus=off  NominalParameters=[2700e6 17000 60]  Reactances1=[ 1.81, 0.3, 0.23, 1.76, 0.65, 0.25, 0.15 ]  Reactances2=[ 1.305, 0.296, 0.252, 0.474, 0.243, 0.18 ]  dAxisTimeConstants=Short-circuit  qAxisTimeConstants=Open-circuit  TimeConstants1="[ 4.4849  0.0681  0.1  ]"  TimeConstants2=[ 8.0, 0.03, 1.0, 0.07 ]  TimeConstants3="[  4.49  0.0681  0.0513  ]"  TimeConstants4=[ 8.0, 0.03, 0.3371, 0.0295 ]  TimeConstants5=[ 1.01, 0.053, 0.1 ]  TimeConstants6=[ 1.3201, 0.023, 1.0, 0.07 ]  TimeConstants7=[0.012 0.003 0.003]  TimeConstants8=[ 1.3201, 0.0231, 0.3371, 0.0295 ]  StatorResistance=2.8544e-3  Mechanical=[3.5 0 32]  PolePairs=20  InitialConditions=[0 -81.9543 0.907703 0.907703 0.907703 -8.76021 -128.76 111.24 1.25655]  SetSaturation=off  Saturation=[0.6404,0.7127,0.8441,0.9214,0.9956,1.082,1.19,1.316,1.457;0.7,0.7698,0.8872,0.9466,0.9969,1.046,1.1,1.151,1.201]  LoadFlowParameters=[1,0,0,0,0]  TsPowergui=0  TsBlock=-1  IterativeModel=Trapezoidal non iterative  IterativeDiscreteModel=Trapezoidal non iterative  BusType=PV  Pref=2200e6  Qref=0  Qmin=-inf  Qmax=inf  PLF=0  QLF=0
  MPP7-BMW 330 km : spsDistributedParametersLineLib/Distributed Parameters Line  Phases=3  Length=330  Frequency=60  Resistance=[0.01273 0.3864]/6  Inductance="[0.9337e-3  4.1264e-3]/6"  Capacitance=[12.74e-9 7.751e-9]*6  x1=[-0.00192 1.38989509065807e-07 0 0;-0.00186 1.40148907189762e-07 0 0;-0.0018 1.41236602543144e-07 0 0;-0.00174 1.42252038640913e-07 0 0;-0.00168 1.43194695967198e-07 0 0;-0.00162 1.44064092241093e-07 0 0;-0.00156 1.44859782663398e-07 0 0;-0.0015 1.45581360144192e-07 0 0;-0.00144 1.46228455511102e-07 0 0;-0.00138 1.46800737698181e-07 0 0;-0.00132 1.47297913915288e-07 0 0;-0.00126 1.47719729797884e-07 0 0;-0.0012 1.48065969537168e-07 0 0;-0.00114 1.48336455990492e-07 -132077.727810692 -207582.11422983;-0.00108 1.48531050771989e-07 -127348.938431694 -210516.312840008;-0.00102 1.48649654323373e-07 -122554.994982656 -213342.807414642;-0.00096 1.48692205964875e-07 -117698.350133629 -216060.151866882;-0.0009 1.4865868392629e-07 -112781.488633858 -218666.955953093;-0.00084 1.48549105358111e-07 -107806.92604054 -221161.885984138;-0.00078 1.48363526322759e-07 -102777.207431817 -223543.665507712;-0.00072 1.48102041765898e-07 -97694.906104667 -225811.0759614;-0.00066 1.47764785467858e-07 -92562.6222583596 -227962.957296118;-0.0006 1.47351929975193e-07 -87382.9816641442 -229998.208569611;-0.00054 1.46863686512403e-07 -82158.6343218576 -231915.788509722;-0.00048 1.46300304873863e-07 -76892.2531041349 -233714.716047121;-0.00042 1.45662073296032e-07 -71586.5323889187 -235394.070817238;-0.00036 1.44949318309977e-07 -66244.1866809652 -236952.993631143;-0.0003 1.44162404574319e-07 -60867.949223054 -238390.686915118;-0.00024 1.43301734688665e-07 -55460.5705976098 -239706.415118714;-0.00018 1.42367748987633e-07 -50024.8173194544 -240899.50509107;-0.00012 1.41360925315566e-07 -44563.470420406 -241969.346425311;-6e-05 1.40281778782058e-07 -39079.3240264523 -242915.391770841]  x2=[-0.00192 9.24024719193905e-08 0 0;-0.00186 9.23789280720258e-08 0 0;-0.0018 9.23081214580931e-08 0 0;-0.00174 9.21900883035645e-08 0 0;-0.00168 9.20248889963828e-08 0 0;-0.00162 9.18126080555661e-08 0 0;-0.00156 9.15533540879663e-08 0 0;-0.0015 9.12472597327035e-08 0 0;-0.00144 9.0894481593306e-08 0 0;-0.00138 9.04952001575885e-08 0 0;-0.00132 9.00496197053113e-08 0 0;-0.00126 8.95579682036672e-08 0 0;-0.0012 8.90204971906491e-08 0 0;-0.00114 8.84374816463587e-08 -71122.359287635 -183857.838140937;-0.00108 8.78092198523211e-08 -66945.7512982624 -185419.440441792;-0.00102 8.71360332388793e-08 -62734.8926255105 -186886.17873076;-0.00096 8.64182662207438e-08 -58491.9376224838 -188257.30259743;-0.0009 8.56562860207837e-08 -54219.0570633627 -189532.110549496;-0.00084 8.48504824821492e-08 -49918.437032795 -190709.950371654;-0.00078 8.40012678688202e-08 -45592.2778074546 -191790.219459287;-0.00072 8.31090766546846e-08 -41242.7927303396 -192772.365126769;-0.00066 8.21743653012532e-08 -36872.2070783845 -193655.884890229;-0.0006 8.1197612024126e-08 -32482.756923968 -194440.326724629;-0.00054 8.01793165483279e-08 -28076.6879908969 -195125.289295033;-0.00048 7.91199998526403e-08 -23656.2545054521 -195710.422161932;-0.00042 7.80202039030586e-08 -19223.7180430851 -196195.425960541;-0.00036 7.68804913755124e-08 -14781.3463713537 -196580.052553954;-0.0003 7.57014453679904e-08 -10331.4122896908 -196864.105160098;-0.00024 7.44836691022162e-08 -5876.19246659796 -197047.438452412;-0.00018 7.32277856150294e-08 -1417.96627485968 -197129.958634196;-0.00012 7.1934437439628e-08 3040.98537462583 -197111.6234866;-6e-05 7.0604286276837e-08 7498.38119980273 -196992.442390224]  x3=[-0.00192 1.3211374894777e-09 0 0;-0.00186 1.3235073406108e-09 0 0;-0.0018 1.32520006093283e-09 0 0;-0.00174 1.32621478441681e-09 0 0;-0.00168 1.32655099191145e-09 0 0;-0.00162 1.32620851140678e-09 0 0;-0.00156 1.32518751812217e-09 0 0;-0.0015 1.32348853441663e-09 0 0;-0.00144 1.32111242952163e-09 0 0;-0.00138 1.31806041909633e-09 0 0;-0.00132 1.31433406460567e-09 0 0;-0.00126 1.30993527252145e-09 0 0;-0.0012 1.30486629334699e-09 0 0;-0.00114 1.2991297204657e-09 -2523.17608134747 -7088.36052883462;-0.00108 1.29272848881426e-09 -2362.20935860076 -7143.6160405756;-0.00102 1.28566587338106e-09 -2200.03408589758 -7195.21674635137;-0.00096 1.27794548753068e-09 -2036.73323510409 -7243.13624628739;-0.0009 1.26957128115515e-09 -1872.39035395303 -7287.35002388205;-0.00084 1.2605475386532e-09 -1707.08952329909 -7327.83545854973;-0.00078 1.25087887673824e-09 -1540.91531410164 -7364.57183719399;-0.00072 1.24057024207636e-09 -1373.95274415665 -7397.5403648047;-0.00066 1.22962690875552e-09 -1206.28723460003 -7426.72417407395;-0.0006 1.21805447558728e-09 -1038.00456620456 -7452.10833402565;-0.00054 1.20585886324226e-09 -869.190835492896 -7473.67985765454;-0.00048 1.1930463112211e-09 -699.932410688998 -7491.42770857053;-0.00042 1.17962337466216e-09 -530.315887530527 -7505.34280664515;-0.00036 1.16559692098781e-09 -360.428044964885 -7515.41803265709;-0.0003 1.15097412639092e-09 -190.355800751494 -7521.64823193457;-0.00024 1.13576247216342e-09 -20.1861669930683 -7524.03021699251;-0.00018 1.11996974086868e-09 149.993794381389 -7522.56276916335;-0.00012 1.10360401235985e-09 320.097016159074 -7517.2466392205;-6e-05 1.08667365964604e-09 490.036470388579 -7508.08454699428]  x4=[-0.00192 1.94244589740713e-10 0 0;-0.00186 2.14529502909702e-10 0 0;-0.0018 2.34704658820953e-10 0 0;-0.00174 2.54759735491907e-10 0 0;-0.00168 2.74684472374765e-10 0 0;-0.00162 2.94468675605971e-10 0 0;-0.00156 3.14102223221581e-10 0 0;-0.0015 3.3357507033585e-10 0 0;-0.00144 3.52877254280375e-10 0 0;-0.00138 3.71998899701189e-10 0 0;-0.00132 3.90930223611167e-10 0 0;-0.00126 4.09661540395185e-10 0 0;-0.0012 4.28183266765462e-10 0 0;-0.00114 4.46485926664545e-10 -3803.20220745506 -511.583500459863;-0.00108 4.64560156113435e-10 -3790.65813109848 -597.47198974746;-0.00102 4.82396708002373e-10 -3776.17468399871 -683.054801325088;-0.00096 4.9998645682183e-10 -3759.75927615493 -768.288149444958;-0.0009 5.17320403331289e-10 -3741.4203059931 -853.128427151238;-0.00084 5.34389679163423e-10 -3721.16715606923 -937.532228590188;-0.00078 5.5118555136131e-10 -3699.01018826905 -1021.45637121739;-0.00072 5.67699426846383e-10 -3674.96073850671 -1104.85791789073;-0.00066 5.83922856814802e-10 -3649.03111092507 -1187.69419883785;-0.0006 5.99847541060021e-10 -3621.23457160074 -1269.92283348678;-0.00054 6.15465332219325e-10 -3591.58534175687 -1351.50175214862;-0.00048 6.30768239942175e-10 -3560.09859048728 -1432.38921754118;-0.00042 6.45748434978212e-10 -3526.79042699574 -1512.54384614254;-0.00036 6.60398253182856e-10 -3491.67789235415 -1591.92462936361;-0.0003 6.74710199438415e-10 -3454.77895078405 -1670.49095452892;-0.00024 6.8867695148873e-10 -3416.11248046575 -1748.20262565476;-0.00018 7.02291363685376e-10 -3375.69826387994 -1825.01988401426;-0.00012 7.15546470643509e-10 -3333.5569776866 -1900.90342847859;-6e-05 7.28435490805482e-10 -3289.71018214643 -1975.81443562427]  x5=0.00186628717108595  V1=[7.602e-19 2.561e-08 2.561e-08;377 377 377;2.359 1.029 -0.5418]  V2=[1.596e-23 1.649e-13 1.649e-13;377 377 377;-0.06951 1.06 -0.5113]  I1=[1.208e-21 2.221e-10 2.221e-10;377 377 377;-2.873 2.204 0.633]  I2=[1.433e-21 2.255e-10 2.255e-10;377 377 377;1.006 -0.507 -2.078]  nHarmo=1  Measurements=None  Decoupling=off  VsMag0=0  VrMag0=0  VsAngle0=0  VrAngle0=0  IsMag0=0  IrMag0=0  IsAngle0=0  IrAngle0=0
      settings: LibrarySourceBlock=sps_lib/Power Grid Elements/Distributed Parameters Line
  MPP8 3100 KVA 17KV : spsSynchronousMachinepuStandardLib/Synchronous Machine pu Standard  PresetModel=No  MechanicalLoad=Mechanical power Pm  ShowDetailedParameters=on  RotorType=Salient-pole  Units=per unit standard parameters  MeasurementBus=off  NominalParameters=[3100e6 17000 60]  Reactances1=[ 1.81, 0.3, 0.23, 1.76, 0.65, 0.25, 0.15 ]  Reactances2=[ 1.305, 0.296, 0.252, 0.474, 0.243, 0.18 ]  dAxisTimeConstants=Short-circuit  qAxisTimeConstants=Open-circuit  TimeConstants1="[ 4.4849  0.0681  0.1  ]"  TimeConstants2=[ 8.0, 0.03, 1.0, 0.07 ]  TimeConstants3="[  4.49  0.0681  0.0513  ]"  TimeConstants4=[ 8.0, 0.03, 0.3371, 0.0295 ]  TimeConstants5=[ 1.01, 0.053, 0.1 ]  TimeConstants6=[ 1.3201, 0.023, 1.0, 0.07 ]  TimeConstants7=[0.012 0.003 0.003]  TimeConstants8=[ 1.3201, 0.0231, 0.3371, 0.0295 ]  StatorResistance=2.8544e-3  Mechanical=[3.5 0 32]  PolePairs=20  InitialConditions=[0 -81.9543 0.907703 0.907703 0.907703 -8.76021 -128.76 111.24 1.25655]  SetSaturation=off  Saturation=[0.6404,0.7127,0.8441,0.9214,0.9956,1.082,1.19,1.316,1.457;0.7,0.7698,0.8872,0.9466,0.9969,1.046,1.1,1.151,1.201]  LoadFlowParameters=[1,0,0,0,0]  TsPowergui=0  TsBlock=-1  IterativeModel=Trapezoidal non iterative  IterativeDiscreteModel=Trapezoidal non iterative  BusType=PV  Pref=2900e6  Qref=0  Qmin=-inf  Qmax=inf  PLF=0  QLF=0
  MPP9 4100 MVA 17KV : spsSynchronousMachinepuStandardLib/Synchronous Machine pu Standard  PresetModel=No  MechanicalLoad=Mechanical power Pm  ShowDetailedParameters=on  RotorType=Salient-pole  Units=per unit standard parameters  MeasurementBus=off  NominalParameters="[4100e6  17000   60]"  Reactances1=[ 1.81, 0.3, 0.23, 1.76, 0.65, 0.25, 0.15 ]  Reactances2=[ 1.305, 0.296, 0.252, 0.474, 0.243, 0.18 ]  dAxisTimeConstants=Short-circuit  qAxisTimeConstants=Open-circuit  TimeConstants1="[ 4.4849  0.0681  0.1  ]"  TimeConstants2=[ 8.0, 0.03, 1.0, 0.07 ]  TimeConstants3="[  4.49  0.0681  0.0513  ]"  TimeConstants4=[ 8.0, 0.03, 0.3371, 0.0295 ]  TimeConstants5=[ 1.01, 0.053, 0.1 ]  TimeConstants6=[ 1.3201, 0.023, 1.0, 0.07 ]  TimeConstants7=[0.012 0.003 0.003]  TimeConstants8=[ 1.3201, 0.0231, 0.3371, 0.0295 ]  StatorResistance=2.8544e-3  Mechanical=[3.5 0 32]  PolePairs=20  InitialConditions=[0 -81.9543 0.907703 0.907703 0.907703 -8.76021 -128.76 111.24 1.25655]  SetSaturation=off  Saturation=[0.6404,0.7127,0.8441,0.9214,0.9956,1.082,1.19,1.316,1.457;0.7,0.7698,0.8872,0.9466,0.9969,1.046,1.1,1.151,1.201]  LoadFlowParameters=[1,0,0,0,0]  TsPowergui=0  TsBlock=-1  IterativeModel=Trapezoidal non iterative  IterativeDiscreteModel=Trapezoidal non iterative  BusType=PV  Pref=3500e6  Qref=0  Qmin=-inf  Qmax=inf  PLF=0  QLF=0
  Regulators 7 : Subsystem
  Regulators 8 : Subsystem
  Regulators 9 : Subsystem
  ATL-a : PMIOPort  Side=Right
  ATL-b : PMIOPort  Port=2  Side=Right
  ATL-c : PMIOPort  Port=3  Side=Right
  ORE-a : PMIOPort  Port=4  Side=Left
  ORE-b : PMIOPort  Port=5  Side=Left
  ORE-c : PMIOPort  Port=6  Side=Left
  wires:
  Regulators 8/2(Vf) -> MPP8 3100 KVA 17KV/2
  MPP8 3100 KVA 17KV/1 -> Regulators 8/1(m)
  Regulators 8/1(Pm) -> MPP8 3100 KVA 17KV/1
  Regulators 7/1(Pm) -> MPP7 2700 MVA 17KV/1
  Regulators 7/2(Vf) -> MPP7 2700 MVA 17KV/2
  Regulators 9/1(Pm) -> MPP9 4100 MVA 17KV/1
  Regulators 9/2(Vf) -> MPP9 4100 MVA 17KV/2
  MPP9 4100 MVA 17KV/1 -> Regulators 9/1(m)
  MPP7 2700 MVA 17KV/1 -> Regulators 7/1(m)
  connections:
  ATL-c/RConn1 -- ATL-CAD 447 km/RConn3
  1320 MVar/LConn2 -- MPP7-BMW 330 km/RConn2 -- "2700 MVA 17KV :650KV Transformer "/LConn2
  1320 MVar/LConn1 -- MPP7-BMW 330 km/RConn1 -- Load Flow Bus1/LConn1 -- "2700 MVA 17KV :650KV Transformer "/LConn1
  Cs FER/RConn3 -- FER-LTN 78 km/LConn3 -- 990 Mvar/LConn3
  MPP8 3100 KVA 17KV/RConn2 -- "3100 MVA 17KV :650KV Transformer "/RConn2 -- 155 MW/LConn2
  1320 MVar/LConn3 -- MPP7-BMW 330 km/RConn3 -- "2700 MVA 17KV :650KV Transformer "/LConn3
  Cs FER/LConn3 -- BMW- FER 131 km/RConn3
  "3100 MVA 17KV :650KV Transformer "/RConn3 -- 155 MW/LConn3 -- MPP8 3100 KVA 17KV/RConn3
  Cs FER/RConn2 -- FER-LTN 78 km/LConn2 -- 990 Mvar/LConn2
  ATL-CAD 447 km/RConn1 -- ATL-a/RConn1
  "3100 MVA 17KV :650KV Transformer "/RConn1 -- MPP8 3100 KVA 17KV/RConn1 -- Load Flow Bus2/LConn1 -- 155 MW/LConn1
  Cs FER/RConn1 -- FER-LTN 78 km/LConn1 -- 990 Mvar/LConn1
  Cs FER/LConn2 -- BMW- FER 131 km/RConn2
  Cs FER/LConn1 -- BMW- FER 131 km/RConn1
  ATL-b/RConn1 -- ATL-CAD 447 km/RConn2
  "2700 MVA 17KV :650KV Transformer "/RConn1 -- 135 MW/LConn1 -- MPP7 2700 MVA 17KV/RConn1 -- Load Flow Bus/LConn1
  "2700 MVA 17KV :650KV Transformer "/RConn2 -- 135 MW/LConn2 -- MPP7 2700 MVA 17KV/RConn2
  "2700 MVA 17KV :650KV Transformer "/RConn3 -- 135 MW/LConn3 -- MPP7 2700 MVA 17KV/RConn3
  "4100 MVA 17KV :650KV Transformer "/LConn1 -- LTN 3/RConn1 -- Load Flow Bus6/LConn1
  "4100 MVA 17KV :650KV Transformer "/LConn2 -- LTN 3/RConn2
  "4100 MVA 17KV :650KV Transformer "/LConn3 -- LTN 3/RConn3
  MPP9 4100 MVA 17KV/RConn1 -- Load Flow Bus4/LConn1 -- 205 MW/LConn1 -- "4100 MVA 17KV :650KV Transformer "/RConn1
  MPP9 4100 MVA 17KV/RConn2 -- 205 MW/LConn2 -- "4100 MVA 17KV :650KV Transformer "/RConn2
  MPP9 4100 MVA 17KV/RConn3 -- 205 MW/LConn3 -- "4100 MVA 17KV :650KV Transformer "/RConn3
  BMW- FER 131 km/LConn1 -- BMW- ORE 215 km/LConn1 -- 660 MVar/LConn1 -- CAD 3/RConn1 -- Load Flow Bus3/LConn1 -- "3100 MVA 17KV :650KV Transformer "/LConn1 -- Cs BMW- MPP8/LConn1
  "3100 MVA 17KV :650KV Transformer "/LConn2 -- BMW- ORE 215 km/LConn2 -- 660 MVar/LConn2 -- Cs BMW- MPP8/LConn2 -- BMW- FER 131 km/LConn2 -- CAD 3/RConn2
  BMW- FER 131 km/LConn3 -- 660 MVar/LConn3 -- BMW- ORE 215 km/LConn3 -- Cs BMW- MPP8/LConn3 -- CAD 3/RConn3 -- "3100 MVA 17KV :650KV Transformer "/LConn3
  Cs BMWN/RConn1 -- MPP7-BMW 330 km/LConn1
  Cs BMWN/RConn2 -- MPP7-BMW 330 km/LConn2
  Cs BMWN/RConn3 -- MPP7-BMW 330 km/LConn3
  BMW 1/RConn1 -- Cs BMWN/LConn1
  BMW 1/RConn2 -- Cs BMWN/LConn2
  BMW 1/RConn3 -- Cs BMWN/LConn3
  Cs BMW- MPP8/RConn1 -- BMW 1/LConn1
  Cs BMW- MPP8/RConn2 -- BMW 1/LConn2
  Cs BMW- MPP8/RConn3 -- BMW 1/LConn3
  ATL-CAD 447 km/LConn1 -- 1980 MVar/LConn1 -- CAD 3/LConn1
  ATL-CAD 447 km/LConn2 -- 1980 MVar/LConn2 -- CAD 3/LConn2
  ATL-CAD 447 km/LConn3 -- Load Flow Bus8/LConn1 -- CAD 3/LConn3 -- 1980 MVar/LConn3
  Cs ORED/RConn1 -- ORE-a/RConn1
  Cs ORED/RConn2 -- ORE-b/RConn1
  Cs ORED/RConn3 -- ORE-c/RConn1
  BMW- ORE 215 km/RConn1 -- Load Flow Bus7/LConn1 -- Cs ORED/LConn1
  BMW- ORE 215 km/RConn2 -- Cs ORED/LConn2
  BMW- ORE 215 km/RConn3 -- Cs ORED/LConn3
  Cs LTNN/RConn1 -- FER-LTN 78 km/RConn1
  Cs LTNN/RConn2 -- FER-LTN 78 km/RConn2
  Cs LTNN/RConn3 -- FER-LTN 78 km/RConn3
  LTN 3/LConn1 -- Cs LTNN/LConn1
  LTN 3/LConn2 -- Cs LTNN/LConn2
  LTN 3/LConn3 -- Cs LTNN/LConn3
